simulink model "VMCBike"  (R2018a)
settings: Solver=VariableStepAuto  StartTime=0.0  StopTime=10  RelTol=1e-3
model workspace (MAT data in the model file):
  C = [0  10.3634836401; -1.76836773663  1.48743615413]
  K = [-70.738929  24.0745033117; -7.253891571  1.04480050199]
  M = [4.1001157  0.406766163568; 0.406766163568  0.213717846179]
  v = 2
values from neighbouring files (symbols this model uses):
  A = [0 0 17.1178625208 1.36125414944 0 0 -6.64054658486 7.75016773723 1 0 -1.01196238812 10.2003638625 ... (16 elements, 4x4)]    [torque_state.mat]
  B = [0  0; 0  0; 0.300668380192  -0.5722578891; -0.5722578891  5.76823680457]    [torque_state.mat]
  Csys = [1 0 0 0 0 1 0 0 0 0 1 0 ... (16 elements, 4x4)]    [torque_state.mat]
settings Model: Creator=User  LastModifiedBy=Philip
settings DebuggingCC: LibraryContextMissingDiagnostic=warning
settings SFSimCC: SimUseLocalCustomCode=on
settings RTWCC: RTWUseLocalCustomCode=on

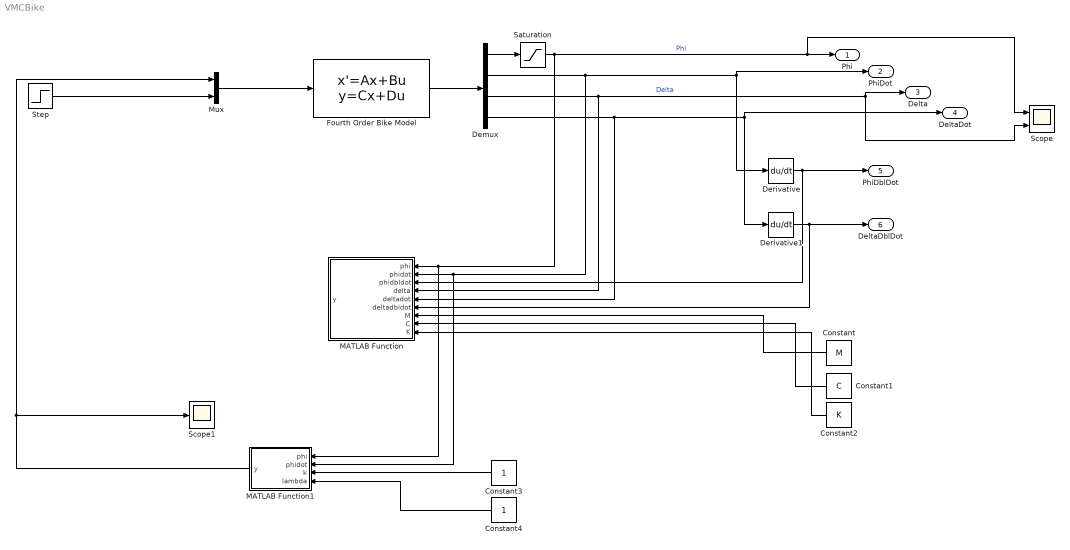
== system VMCBike ==
  Constant : Constant  Value=M
  Constant1 : Constant  Value=C
  Constant2 : Constant  Value=K
  Constant3 : Constant
  Constant4 : Constant
  Demux : Demux
  Derivative : Derivative
  Derivative1 : Derivative
  Fourth Order Bike Model : StateSpace  A=A  B=B  C=Csys  D=zeros(4,2)  InitialCondition=0
  MATLAB Function : MATLAB Function  TreatAsAtomicUnit=on
  MATLAB Function1 : MATLAB Function  TreatAsAtomicUnit=on
  Mux : Mux  Inputs=2
  Saturation : Saturate  UpperLimit=pi/2  LowerLimit=-pi/2
  Scope : Scope  NumInputPorts=2
  Scope1 : Scope
  Step : Step  After=0.01  SampleTime=0
  Phi : Outport
  PhiDot : Outport  Port=2
  Delta : Outport  Port=3
  DeltaDot : Outport  Port=4
  PhiDblDot : Outport  Port=5
  DeltaDblDot : Outport  Port=6
  wires:
  Fourth Order Bike Model/1 -> Demux/1
  Demux/2 -> MATLAB Function1/2(phidot), MATLAB Function/2(phidot), PhiDot/1, Derivative/1
  Demux/3 -> MATLAB Function/4(delta), Delta/1, Scope/2  "Delta"
  Derivative/1 -> MATLAB Function/3(phidbldot), PhiDblDot/1
  Derivative1/1 -> MATLAB Function/6(deltadbldot), DeltaDblDot/1
  Demux/4 -> MATLAB Function/5(deltadot), DeltaDot/1, Derivative1/1
  Mux/1 -> Fourth Order Bike Model/1
  Constant/1 -> MATLAB Function/7(M)
  Constant1/1 -> MATLAB Function/8(C)
  Constant2/1 -> MATLAB Function/9(K)
  Demux/1 -> Saturation/1
  Saturation/1 -> MATLAB Function1/1(phi), MATLAB Function/1(phi), Scope/1, Phi/1  "Phi"
  Step/1 -> Mux/2
  MATLAB Function1/1(y) -> Scope1/1, Mux/1
  Constant3/1 -> MATLAB Function1/3(k)
  Constant4/1 -> MATLAB Function1/4(lambda)

== matlab function VMCBike/MATLAB Function1 ==
  data: phi input; y output; phidot input; k input; lambda input
function y = fcn(phi, phidot, k, lambda)

l = 1;

y = -l * cos(phi/2) * (2 * l * k * sin(phi/2) + lambda * l * phidot * cos(phi/2));

== matlab function VMCBike/MATLAB Function ==
  data: phi input; y output; phidot input; phidbldot input; delta input; deltadot input; deltadbldot input; M input; C input; K input
function y = fcn(phi, phidot, phidbldot, delta, deltadot, deltadbldot, M, C, K)

y = (M(2,1) - M(1,1)) * phidbldot + (M(2,2) - M(1,2)) * deltadbldot + ...
    (C(2,1) - C(1,1)) * phidot    + (C(2,2) - C(1,2)) * deltadot    + ...
    (K(2,1) - K(1,1)) * phi       + (K(2,2) - K(1,2)) * delta;
